simulink model "func2_d"  (R2020a)
settings: Solver=VariableStepAuto  StartTime=0.0  StopTime=10.0  RelTol=1e-3  EnableMultiTasking=on
undefined symbols (not defined in the file or in its folder): S, vsva2197, xcvc1902
libraries: ModelComposer x2, dspsigattribs x1, fixedpoint_complex_2_lib x1
settings Model: Creator=abehbood  LastModifiedBy=viswanad
settings DataIOCC: ReturnWorkspaceOutputs=off
settings OptimizationCC: LifeSpan=inf
settings DebuggingCC: SFUnexpectedBacktrackingDiag=warning  SFNoUnconditionalDefaultTransitionDiag=warning  ArithmeticOperatorsInVariantConditions=warning
settings SFSimCC: SimUseLocalCustomCode=off  CustomCodeUndefinedFunction=UseInterfaceOnly
settings RTWCC: RTWUseLocalCustomCode=off
settings CodeAppCC: StateflowObjectComments=on
settings GRTTargetCC: TargetLangStandard=C89/C90 (ANSI)
settings ConfigComp: CovMetricSettings=dw  CovHtmlReporting=on  CovSaveCumulativeToWorkspaceVar=on  CovSaveSingleToWorkspaceVar=on  CovExternalEMLEnable=off

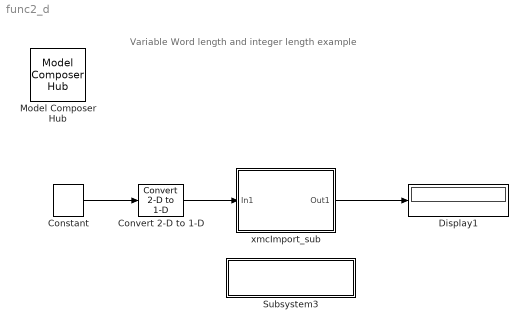
== system func2_d ==
  note: Variable Word length and integer length example
  Constant : ModelComposer/Constant  Value=[1 2 3 4 5 6]  VectorParams1D=off  SampleTime=1.0  OutDataType=fixed  TypeExp=''  Signedness=Signed  WordLength=16  FractionalLength=5  RoundingMode=Truncation to minus infinity  OverflowMode=Wrap around
  Convert 2-D to 1-D : dspsigattribs/Convert 2-D to 1-D
      settings: SourceProductBaseCode=DS
  Display1 : Display
  Model Composer Hub : ModelComposer/Model Composer Hub  CodeGeneration=off  SubsystemName=xmcImport_sub  TargetDirectory=./code  ExportType=IP Catalog  IpVendor=xilinx.com  IpLibrary=hls  IpVersion=1.0  IpHWLanguage=Verilog  AieCompilerOptions={}  CreateTestbench=off  TestbenchStackSize=10  RunAieSim=off  AieSimTimeout=50000  RunAieSimProfiling=off  LaunchVitisAnalyzer=off  PlotOutput=off  RunX86Sim=off  X86SimTimeout=10  GenHwImage=off  PlatformType=Not Specified  ProjDevice=xcvc1902-vsva2197-2MP-e-S  ProjDevicePart=xcvc1902-vsva2197-2MP-e-S  SamplePeriod=-1  ClockFrequency=200  DataPathParallelism=1
  Subsystem3 : Subsystem
      settings: OpenFcn=xmcOpenFileEx
      mask Display: disp(sprintf('Double Click to open\nthe main header file'))
  xmcImport_sub : Subsystem
  wires:
  Constant/1 -> Convert 2-D to 1-D/1
  Convert 2-D to 1-D/1 -> xmcImport_sub/1(In1)
  xmcImport_sub/1(Out1) -> Display1/1

== system func2_d/Subsystem3 ==

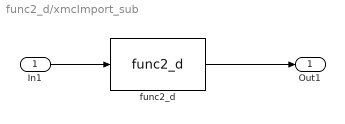
== system func2_d/xmcImport_sub ==
  In1 : Inport
  func2_d : fixedpoint_complex_2_lib/func2_d  LibraryFunction=func2_d  IncludeFiles={'func2_d.h'}  SourceFiles={}  IncludeDirectories={}  TemplateParams={'int WordLen'; 'int IntLen'; 'int SIZE'}  FunctionParamTypes={xmcDataType('void'); xmcDataType('const ap_fixed<WordLen, IntLen>'); xmcDataType('ap_fixed<WordLen + 1, IntLen> &')}  FunctionParamPassbys={0.000000000000000000e+00; 0.000000000000000000e+00; 1.000000000000000000e+00}  FunctionParamDimensions={'1'; '[SIZE]'; '1'}  FunctionParamNames={'return'; 'in1'; 'out'}  FunctionParamDir={0.000000000000000000e+00; 1.000000000000000000e+00; 2.000000000000000000e+00}  FunctionParamSupportsStreaming={false; false; false}  BufferDepth={'0'}  FunctionParamValues={'0'; '0'; '0'}  ThroughputFactors={''}
  Out1 : Outport
  wires:
  func2_d/1 -> Out1/1
  In1/1 -> func2_d/1
